simulink model "PA_Heading_Hold"  (Simulink 8.7)
settings: Solver=ode4  StartTime=0.0  StopTime=300  FixedStep=0.01  RelTol=1e-3
undefined symbols (not defined in the file or in its folder): degtorad, Ue
libraries: xpcutilitieslib x2, instrumentlib x2, xpcobsoletelib x2, sldrtlib x1
settings Model: Creator=Marcelo Henrique  LastModifiedBy=Pegasus
settings DataIOCC: MaxDataPoints=10000
settings DebuggingCC: AlgebraicLoopMsg=none  StateNameClashWarn=warning

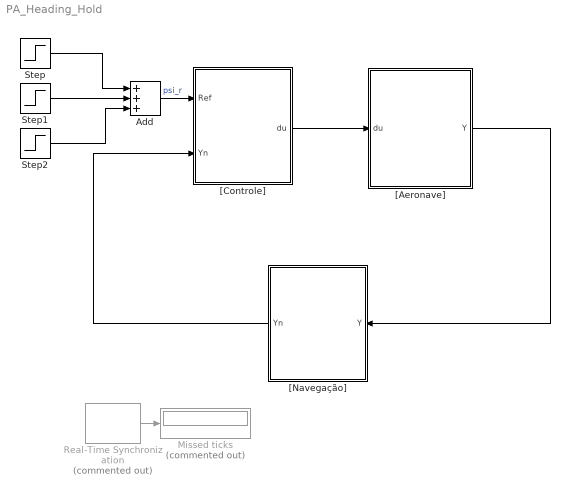
== system PA_Heading_Hold ==
  Add : Sum  Inputs=+++
  Missed ticks : Display  Commented=on
  Real-Time Synchronization : sldrtlib/Real-Time Synchronization  Commented=on  SampleTime=0.01  MaxMissedTicks=inf  ShowMissedTicks=on  YieldWhenWaiting=on
  Step : Step  Time=50  After=degtorad(45)  SampleTime=0
  Step1 : Step  Time=150  After=degtorad(-90)  SampleTime=0
  Step2 : Step  Time=250  After=degtorad(45)  SampleTime=0
  "[Aeronave]" : Subsystem
  "[Controle]" : Subsystem
  "[Navegação]" : Subsystem
  wires:
  "[Navegação]"/1(Yn) -> "[Controle]"/2(Yn)
  "[Controle]"/1(du) -> "[Aeronave]"/1(du)
  "[Aeronave]"/1(Y) -> "[Navegação]"/1(Y)
  Real-Time Synchronization/1 -> Missed ticks/1
  Step/1 -> Add/1
  Add/1 -> "[Controle]"/1(Ref)  "psi_r"
  Step1/1 -> Add/2
  Step2/1 -> Add/3

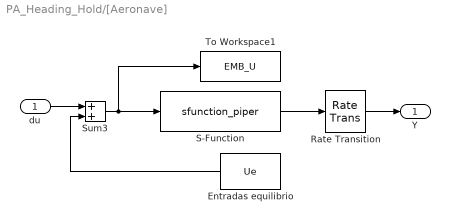
== system PA_Heading_Hold/[Aeronave] ==
  du : Inport
  Entradas equilibrio : Constant  Value=Ue
  Rate Transition : RateTransition  OutPortSampleTime=0.01
  S-Function : S-Function  FunctionName=sfunction_piper  Parameters=par_gen,par_aero,par_prop, Xe  SFunctionDeploymentMode=off  EnableBusSupport=off
  Sum3 : Sum
  To Workspace1 : ToWorkspace  VariableName=EMB_U  SaveFormat=Timeseries  SampleTime=-1
  Y : Outport
  wires:
  S-Function/1 -> Rate Transition/1
  du/1 -> Sum3/1
  Entradas equilibrio/1 -> Sum3/2
  Sum3/1 -> To Workspace1/1, S-Function/1
  Rate Transition/1 -> Y/1

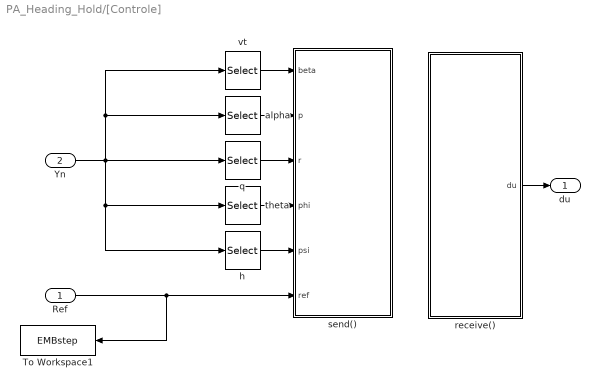
== system PA_Heading_Hold/[Controle] ==
  Ref : Inport
  Yn : Inport  Port=2
  To Workspace1 : ToWorkspace  VariableName=EMBstep  SaveFormat=Timeseries  SampleTime=-1
  alpha : Selector  InputPortWidth=5  IndexOptions=Index vector (dialog)  Indices=[2]  OutputSizes=1
  h : Selector  InputPortWidth=5  IndexOptions=Index vector (dialog)  Indices=[5]  OutputSizes=1
  q : Selector  InputPortWidth=5  IndexOptions=Index vector (dialog)  Indices=[3]  OutputSizes=1
  receive() : Subsystem
  send() : Subsystem
  theta : Selector  InputPortWidth=5  IndexOptions=Index vector (dialog)  Indices=[4]  OutputSizes=1
  vt : Selector  InputPortWidth=5  IndexOptions=Index vector (dialog)  Indices=[1]  OutputSizes=1
  du : Outport
  wires:
  Ref/1 -> To Workspace1/1, send()/6(ref)
  receive()/1(du) -> du/1
  vt/1 -> send()/1(beta)
  alpha/1 -> send()/2(p)
  q/1 -> send()/3(r)
  theta/1 -> send()/4(phi)
  h/1 -> send()/5(psi)
  Yn/1 -> h/1, theta/1, alpha/1, vt/1, q/1

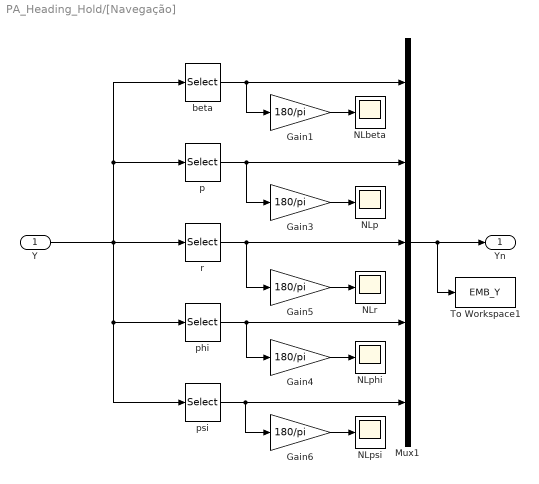
== system PA_Heading_Hold/[Navegação] ==
  Y : Inport
  Gain{1,3..6} (5 alike) : Gain  Gain=180/pi
  Mux1 : Mux  Inputs=5
  NLbeta : Scope
  NLp : Scope
  NLphi : Scope
  NLpsi : Scope
  NLr : Scope
  To Workspace1 : ToWorkspace  VariableName=EMB_Y  SaveFormat=Timeseries  SampleTime=-1
  beta : Selector  InputPortWidth=12  IndexOptions=Index vector (dialog)  Indices=[3]  OutputSizes=1
  p : Selector  InputPortWidth=12  IndexOptions=Index vector (dialog)  Indices=[4]  OutputSizes=1
  phi : Selector  InputPortWidth=12  IndexOptions=Index vector (dialog)  Indices=[7]  OutputSizes=1
  psi : Selector  InputPortWidth=12  IndexOptions=Index vector (dialog)  Indices=[9]  OutputSizes=1
  r : Selector  InputPortWidth=12  IndexOptions=Index vector (dialog)  Indices=[6]  OutputSizes=1
  Yn : Outport
  wires:
  Mux1/1 -> Yn/1, To Workspace1/1
  r/1 -> Mux1/3, Gain5/1
  Gain5/1 -> NLr/1
  p/1 -> Mux1/2, Gain3/1
  Gain3/1 -> NLp/1
  psi/1 -> Mux1/5, Gain6/1
  phi/1 -> Mux1/4, Gain4/1
  Gain4/1 -> NLphi/1
  Y/1 -> phi/1, psi/1, r/1, p/1, beta/1
  Gain6/1 -> NLpsi/1
  beta/1 -> Gain1/1, Mux1/1
  Gain1/1 -> NLbeta/1

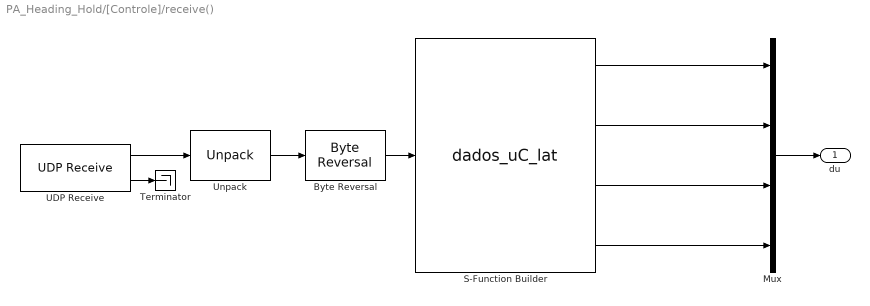
== system PA_Heading_Hold/[Controle]/receive() ==
  Byte Reversal : xpcutilitieslib/Byte Reversal   numInp=1
  Mux : Mux
  S-Function Builder : S-Function  InitFcn=try, set_param(gcb,'FunctionName','dados_uC_lat'), end  FunctionName=dados_uC_lat  SFunctionModules=dados_uC_lat_wrapper  WizardData=DataTag0  SFunctionDeploymentMode=off  EnableBusSupport=off  mask(S-Function Builder){}
      mask help: Simulink:masks:SFunctionBuilder_MD
      mask init:
      | val = [[.9  0.75 0.75 1 1 .9 .9 1]',[1 1 0.75 0.75 .9 .9 1 .9]'];try , sys = get_param(gcb,'SfunBuilderFcnName');if isempty(sys), sys = get_param(gcb,'FunctionName'); end,catch, sys = get_param(gcb,'FunctionName'); end
      settings: CopyFcn=set_param(gcbh,'LinkStatus','none')  PreSaveFcn=try, set_param(gcb,'FunctionName','dados_uC_lat'), end  OpenFcn=sfunctionwizard(gcbh)
      mask Display: plot(val(:,1),val(:,2)),disp(sys), port_label('input',1,'control'), port_label('output',1,'ut'), port_label('output',2,'ue'), port_label('output',3,'ua'), port_label('output',4,'ur')
  Terminator : Terminator
  UDP Receive : instrumentlib/UDP Receive  Host=192.168.1.101  Port=45004  LocalPort=45000  DataSize=16  EnableBlockingMode=off  Timeout=10  SampleTime=0.01  DataType=uint8  ByteOrder=BigEndian
  Unpack : xpcobsoletelib/Utilities/Unpack   dimensions={[1 16]}  datatypes={'uint8'}  byteAlign=1
  du : Outport
  wires:
  UDP Receive/1 -> Unpack/1
  Unpack/1 -> Byte Reversal/1
  Byte Reversal/1 -> S-Function Builder/1
  UDP Receive/2 -> Terminator/1
  S-Function Builder/4 -> Mux/4
  S-Function Builder/1 -> Mux/1
  Mux/1 -> du/1
  S-Function Builder/2 -> Mux/2
  S-Function Builder/3 -> Mux/3

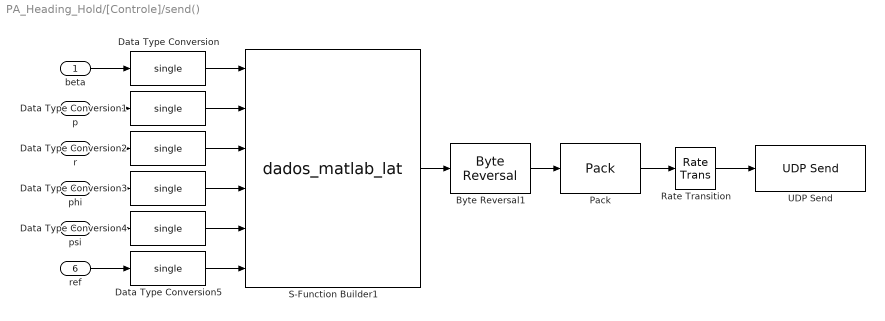
== system PA_Heading_Hold/[Controle]/send() ==
  beta : Inport
  p : Inport  Port=2
  r : Inport  Port=3
  phi : Inport  Port=4
  psi : Inport  Port=5
  ref : Inport  Port=6
  Byte Reversal1 : xpcutilitieslib/Byte Reversal   numInp=1
  Data Type Conversion{,1..5} (6 alike) : DataTypeConversion  OutDataTypeStr=single
  Pack : xpcobsoletelib/Utilities/Pack   datatypes={'uint8'}  byteAlign=1
  Rate Transition : RateTransition  OutPortSampleTime=0.01
  S-Function Builder1 : S-Function  InitFcn=try, set_param(gcb,'FunctionName','dados_matlab_lat'), end  FunctionName=dados_matlab_lat  SFunctionModules=dados_matlab_lat_wrapper  WizardData=DataTag1  SFunctionDeploymentMode=off  EnableBusSupport=off  mask(S-Function Builder){}
      mask help: Simulink:masks:SFunctionBuilder_MD
      mask init: same as PA_Heading_Hold/[Controle]/receive()/S-Function Builder
      settings: CopyFcn=set_param(gcbh,'LinkStatus','none')  PreSaveFcn=try, set_param(gcb,'FunctionName','dados_matlab_lat'), end  OpenFcn=sfunctionwizard(gcbh)
      mask Display: plot(val(:,1),val(:,2)),disp(sys), port_label('input',1,'beta'), port_label('input',2,'p'), port_label('input',3,'r'), port_label('input',4,'phi'), port_label('input',5,'psi'), port_label('input',6,'ref'), port_label('output',1,'data')
  UDP Send : instrumentlib/UDP Send  Host=192.168.1.101  Port=45004  LocalPort=45001  EnableBlockingMode=on  ByteOrder=BigEndian
  wires:
  Byte Reversal1/1 -> Pack/1
  beta/1 -> Data Type Conversion/1
  S-Function Builder1/1 -> Byte Reversal1/1
  p/1 -> Data Type Conversion1/1
  r/1 -> Data Type Conversion2/1
  phi/1 -> Data Type Conversion3/1
  psi/1 -> Data Type Conversion4/1
  Data Type Conversion/1 -> S-Function Builder1/1
  Data Type Conversion1/1 -> S-Function Builder1/2
  Data Type Conversion2/1 -> S-Function Builder1/3
  ref/1 -> Data Type Conversion5/1
  Data Type Conversion5/1 -> S-Function Builder1/6
  Data Type Conversion4/1 -> S-Function Builder1/5
  Data Type Conversion3/1 -> S-Function Builder1/4
  Pack/1 -> Rate Transition/1
  Rate Transition/1 -> UDP Send/1
